simulink model "lpf_sim"  (R2012b)
settings: Solver=FixedStepDiscrete  StartTime=0.0  StopTime=10.0  FixedStep=0.1  RelTol=1e-3
libraries: simulink x1
settings Model: Creator=Krish  LastModifiedBy=Krish

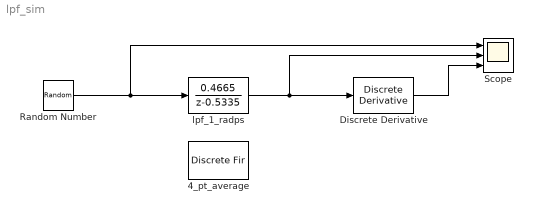
== system lpf_sim ==
  4_pt_average : DiscreteFir  Coefficients=[0.25 0.25 0.25 0.25]  InitialStates=1
  Discrete Derivative : simulink/Discrete/Discrete Derivative  gainval=1.0  ICPrevScaledInput=0.0  InputProcessing=Inherited  OutMin=[]  OutMax=[]  OutDataType=fixdt(1, 16)  OutScaling=2^-10  DoSatur=off
  Random Number : RandomNumber  Mean=1  Variance=0.1  SampleTime=0.1
  Scope : Scope  NumInputPorts=3
      settings: YMin=-5~-5~-5  YMax=5~5~5
  lpf_1_radps : DiscreteTransferFcn  Numerator=[0.4665]  Denominator=[1 -0.5335]  InitialStates=1
  wires:
  Random Number/1 -> lpf_1_radps/1, Scope/1
  lpf_1_radps/1 -> Scope/2, Discrete Derivative/1
  Discrete Derivative/1 -> Scope/3
